simulink model "DAC"  (Simulink 8.8)
settings: Solver=ode3  StartTime=0.0  StopTime=3*T0  FixedStep=Te  RelTol=1e-3  EnableMultiTasking=on
InitFcn:
  | DAC_InitFcn()
StopFcn:
  | DAC_StopFcn()
values from neighbouring files (symbols this model uses):
  F0 = 1e3    (= 1000)    [DAC_InitFcn.m]
  SD = 100    [DAC_InitFcn.m]
  Tau = 2*pi/Fe    (= 0.000628318530718)    [DAC_InitFcn.m]
  W = [32 16 8 4 1 1 1 1 1]'    [DAC_InitFcn.m]    (also in DAC_SubFunction.m = 2.^NMSB')
settings Model: LogicAnalyzerSignalOrdering=5da97608-3139-466b-9f8d-1a0159a4ac02,36d8ee5a-273f-4e98-a89d-e1c511cae97e,31d6a21e-e3d1-410a-9d5d-ac2a4e33df0d,2c1a629a-a9ea-40c1-9ca8-6c9ddaa09610  SuppressorTable=22 serialization::archive 11 0 3 0 0 0 0 0  Creator=F555267  LastModifiedBy=liuqh  SimulationMode=accelerator
settings Model: LogicAnalyzerGraphicalSettings=|
  | {
  |   "cursors" : {
  |     "activeCursor" : 0,
  |     "lockedCursors" : [
  | 
  |     ],
  |     "startingCursor" : 0,
  |     "times" : [
  |       0.001242
  |     ]
  |   },
  |   "global" : {
  |   },
  |   "panels" : [
  |     {
  |       "height" : 100,
  |       "startingTrace" : 0,
  |       "traces" : [
  |         {
  |           "signalId" : "5da97608-3139-466b-9f8d-1a0159a4ac02",
  |           "type" : "wave"
  |         },
  |         {
  |           "expandChannels" : true,
  |           "signalId" : "36d8ee5a-273f-4e98-a89d-e1c511cae97e",
  |           "subWaves" : {
  |           },
  |           "type" : "wave"
  |         },
  |         {
  |           "signalId" : "31d6a21e-e3d1-410a-9d5d-ac2a4e33df0d",
  |           "type" : "wave"
  |         },
  |         {
  |           "signalId" : "2c1a629a-a9ea-40c1-9ca8-6c9ddaa09610",
  |           "type" : "wave"
  |         }
  |       ],
  |       "yOffset" : 0
  |     }
  |   ],
  |   "timeAxis" : {
  |     "pixelsPerSecond" : 283295.45454545453
  |   }
  | }
settings OptimizationCC: ExpressionDepthLimit=2147483647
settings DebuggingCC: SolverPrmCheckMsg=warning
settings ConfigComp: CovSFcnEnable=off

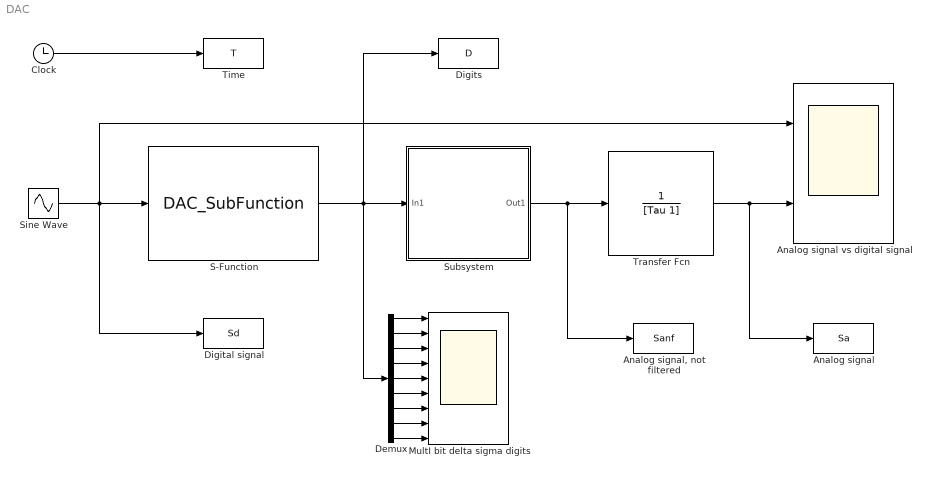
== system DAC ==
  Analog signal : ToWorkspace  VariableName=Sa  SampleTime=-1
      settings: Save2DSignal=2-D array (concatenate along first dimension)
  Analog signal vs digital signal : Scope  NumInputPorts=2
  "Analog signal, not filtered" : ToWorkspace  VariableName=Sanf  SampleTime=-1
      settings: Save2DSignal=2-D array (concatenate along first dimension)
  Clock : Clock
  Demux : Demux  Outputs=9
  Digital signal : ToWorkspace  VariableName=Sd  SampleTime=-1
  Digits : ToWorkspace  VariableName=D  SampleTime=-1
      settings: Save2DSignal=2-D array (concatenate along first dimension)
  MultI bit delta sigma digits : Scope  NumInputPorts=9
  S-Function : S-Function  FunctionName=DAC_SubFunction  SFunctionDeploymentMode=off  EnableBusSupport=off
      mask Display: disp('Multi bit delta sigma DAC')
  Sine Wave : Sin  Amplitude=SD  Frequency=2*pi*F0  SampleTime=0
  Subsystem : Subsystem
      mask Display: disp('Summation')
  Time : ToWorkspace  VariableName=T  SampleTime=-1
  Transfer Fcn : TransferFcn  Numerator=1  Denominator=[Tau 1]
      mask Display: disp('Low pass filter')
  wires:
  S-Function/1 -> Digits/1, Demux/1, Subsystem/1(In1)
  Clock/1 -> Time/1
  Sine Wave/1 -> Digital signal/1, S-Function/1, Analog signal vs digital signal/1
  Demux/1 -> MultI bit delta sigma digits/1
  Demux/2 -> MultI bit delta sigma digits/2
  Demux/3 -> MultI bit delta sigma digits/3
  Demux/4 -> MultI bit delta sigma digits/4
  Demux/5 -> MultI bit delta sigma digits/5
  Demux/6 -> MultI bit delta sigma digits/6
  Demux/7 -> MultI bit delta sigma digits/7
  Demux/8 -> MultI bit delta sigma digits/8
  Demux/9 -> MultI bit delta sigma digits/9
  Transfer Fcn/1 -> Analog signal/1, Analog signal vs digital signal/2
  Subsystem/1(Out1) -> "Analog signal, not filtered"/1, Transfer Fcn/1

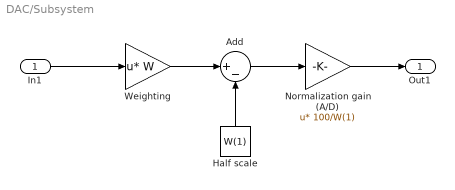
== system DAC/Subsystem ==
  In1 : Inport
  Add : Sum  Inputs=|+-
  Half scale : Constant  Value=W(1)
  Normalization gain (A/D) : Gain  Gain=100/W(1)  Multiplication=Matrix(u*K)
  Weighting : Gain  Gain=W  Multiplication=Matrix(u*K)
  Out1 : Outport
  wires:
  In1/1 -> Weighting/1
  Weighting/1 -> Add/1
  Add/1 -> Normalization gain (A/D)/1
  Half scale/1 -> Add/2
  Normalization gain (A/D)/1 -> Out1/1
